simulink model "Problem_1_Part_A"  (R2018b)
settings: Solver=FixedStepAuto  StartTime=0.0  StopTime=200  FixedStep=0.01  RelTol=1e-3
InitFcn:
  | Initial_Data
StopFcn:
  | Plots_Problme_1_Part_A
values from neighbouring files (symbols this model uses):
  desired_distance = 5    [Initial_Data.m]
  K = 5    [Initial_Data.m]
  Psi0 = 0    [Initial_Data.m]
  V = 30    [Initial_Data.m]
  X0 = 500    [Initial_Data.m]
  Y0 = 0    [Initial_Data.m]
libraries: vrlib x2, simulink x1, simulink_extras x1
settings Model: Creator=User  LastModifiedBy=User

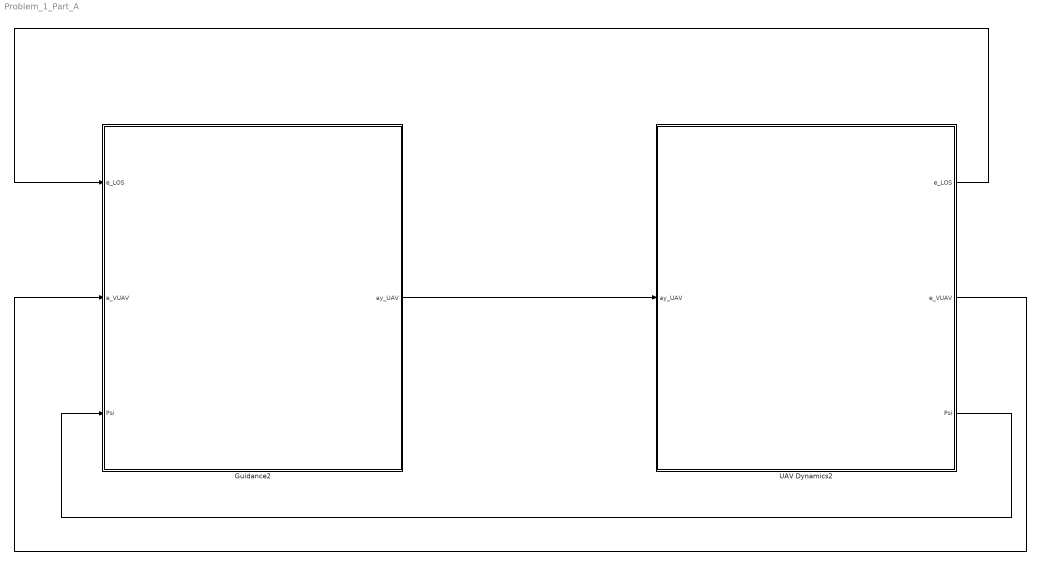
== system Problem_1_Part_A ==
  Guidance2 : Subsystem
  UAV Dynamics2 : Subsystem
  wires:
  UAV Dynamics2/2(e_VUAV) -> Guidance2/2(e_VUAV)
  UAV Dynamics2/1(e_LOS) -> Guidance2/1(e_LOS)
  UAV Dynamics2/3(Psi) -> Guidance2/3(Psi)
  Guidance2/1(ay_UAV) -> UAV Dynamics2/1(ay_UAV)

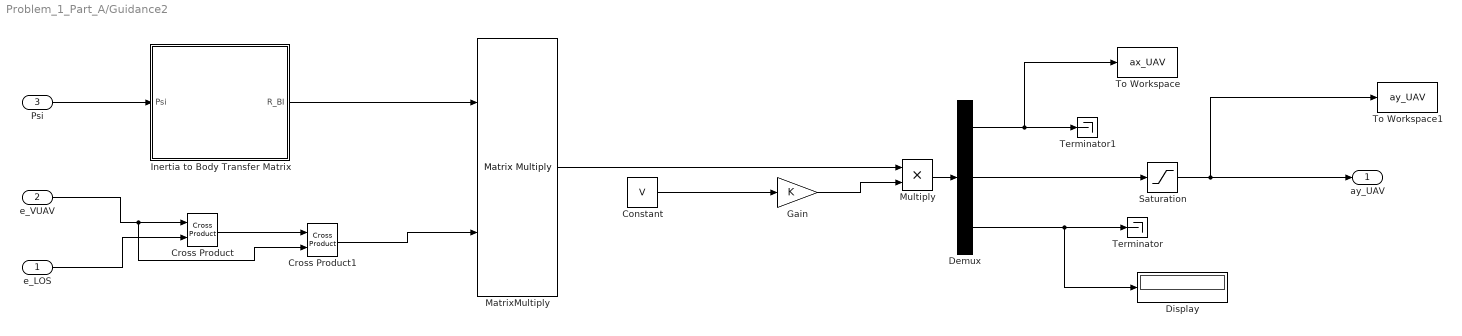
== system Problem_1_Part_A/Guidance2 ==
  e_LOS : Inport
  e_VUAV : Inport  Port=2
  Psi : Inport  Port=3
  Constant : Constant  Value=V
  Cross Product : vrlib/Utilities/Cross Product
      settings: SourceProductBaseCode=VR
  Cross Product1 : vrlib/Utilities/Cross Product
      settings: SourceProductBaseCode=VR
  Demux : Demux  Outputs=3
  Display : Display
  Gain : Gain  Gain=K
  Inertia to Body Transfer Matrix : MATLAB Function  TreatAsAtomicUnit=on
  MatrixMultiply : Product  Multiplication=Matrix(*)
  Multiply : Product
  Saturation : Saturate  UpperLimit=10  LowerLimit=-10
  Terminator : Terminator
  Terminator1 : Terminator
  To Workspace : ToWorkspace  VariableName=ax_UAV  SaveFormat=Timeseries  SampleTime=-1
  To Workspace1 : ToWorkspace  VariableName=ay_UAV  SaveFormat=Timeseries  SampleTime=-1
  ay_UAV : Outport
  wires:
  e_VUAV/1 -> Cross Product/1, Cross Product1/2
  e_LOS/1 -> Cross Product/2
  Psi/1 -> Inertia to Body Transfer Matrix/1(Psi)
  Inertia to Body Transfer Matrix/1(R_BI) -> MatrixMultiply/1
  Cross Product/1 -> Cross Product1/1
  Cross Product1/1 -> MatrixMultiply/2
  Demux/2 -> Saturation/1
  Demux/3 -> Terminator/1, Display/1
  Constant/1 -> Gain/1
  MatrixMultiply/1 -> Multiply/1
  Gain/1 -> Multiply/2
  Multiply/1 -> Demux/1
  Demux/1 -> To Workspace/1, Terminator1/1
  Saturation/1 -> To Workspace1/1, ay_UAV/1

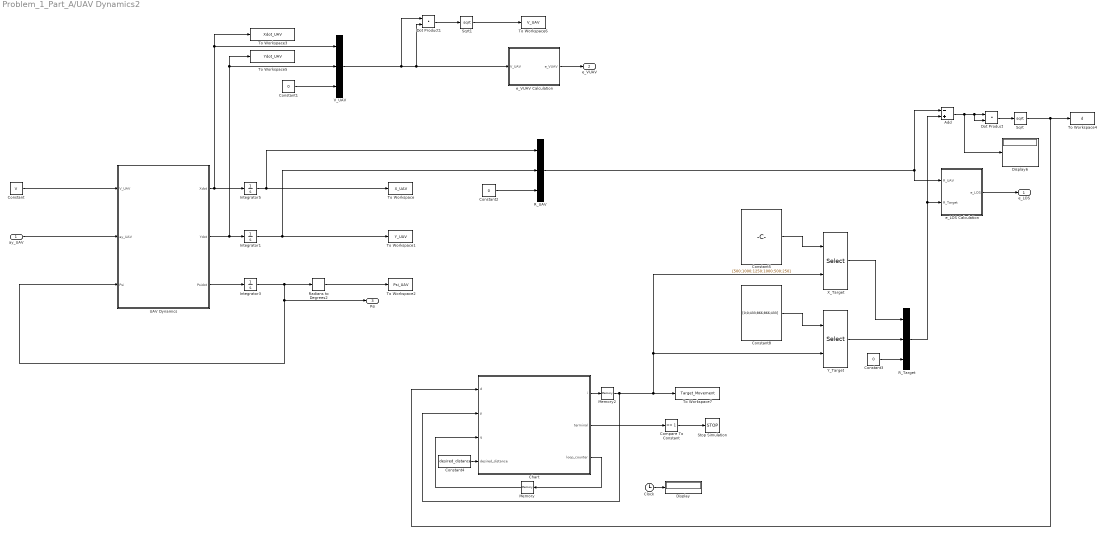
== system Problem_1_Part_A/UAV Dynamics2 ==
  ay_UAV : Inport
  Add : Sum  Inputs=-+
  Chart : Stateflow chart  TreatAsAtomicUnit=on
  Clock : Clock
  Compare To Constant : simulink/Logic and Bit Operations/Compare To Constant  relop===  const=1  OutDataTypeStr=boolean
  Constant : Constant  Value=V
  Constant1 : Constant  Value=0
  Constant2 : Constant  Value=0
  Constant3 : Constant  Value=0
  Constant4 : Constant  Value=desired_distance
  Constant5 : Constant  Value=[500;1000;1250;1000;500;250]  VectorParams1D=off
  Constant8 : Constant  Value=[0;0;433;866;866;433]  VectorParams1D=off
  Display : Display
  Display6 : Display
  Dot Product : DotProduct  InputSameDT=on  OutDataTypeStr=Inherit: Inherit via internal rule
  Dot Product1 : DotProduct  InputSameDT=on  OutDataTypeStr=Inherit: Inherit via internal rule
  Integrator1 : Integrator  InitialCondition=Y0
  Integrator3 : Integrator  InitialCondition=Psi0*pi/180
  Integrator5 : Integrator  InitialCondition=X0
  Memory : Memory  InitialCondition=1
  Memory2 : Memory  InitialCondition=2
  R_Target : Mux  Inputs=3
  R_UAV : Mux  Inputs=3
  Radians to Degrees2 : simulink_extras/Transformations/Radians to Degrees
  Sqrt : Sqrt  SaturateOnIntegerOverflow=on
  Sqrt1 : Sqrt  SaturateOnIntegerOverflow=on
  Stop Simulation : Stop
  To Workspace : ToWorkspace  VariableName=X_UAV  SaveFormat=Timeseries  SampleTime=-1
  To Workspace1 : ToWorkspace  VariableName=Y_UAV  SaveFormat=Timeseries  SampleTime=-1
  To Workspace2 : ToWorkspace  VariableName=Psi_UAV  SaveFormat=Timeseries  SampleTime=-1
  To Workspace3 : ToWorkspace  VariableName=Xdot_UAV  SaveFormat=Timeseries  SampleTime=-1
  To Workspace4 : ToWorkspace  VariableName=d  SaveFormat=Timeseries  SampleTime=-1
  To Workspace5 : ToWorkspace  VariableName=Ydot_UAV  SaveFormat=Timeseries  SampleTime=-1
  To Workspace6 : ToWorkspace  VariableName=V_UAV  SaveFormat=Timeseries  SampleTime=-1
  To Workspace7 : ToWorkspace  VariableName=Target_Movement  SaveFormat=Timeseries  SampleTime=-1
  UAV Dynamics : MATLAB Function  TreatAsAtomicUnit=on
  V_UAV : Mux  Inputs=3
  X_Target : Selector  InputPortWidth=6  IndexOptions=Index vector (port)  Indices=1  OutputSizes=2
  Y_Target : Selector  InputPortWidth=6  IndexOptions=Index vector (port)  Indices=1  OutputSizes=2
  e_LOS Calculation : MATLAB Function  TreatAsAtomicUnit=on
  e_VUAV Calculation : MATLAB Function  TreatAsAtomicUnit=on
  e_LOS : Outport
  e_VUAV : Outport  Port=2
  Psi : Outport  Port=3
  wires:
  UAV Dynamics/1(Xdot) -> Integrator5/1, To Workspace3/1, V_UAV/1
  Integrator1/1 -> To Workspace1/1, R_UAV/2
  UAV Dynamics/3(Psidot) -> Integrator3/1
  Constant2/1 -> R_UAV/3
  Constant3/1 -> R_Target/3
  R_Target/1 -> Add/2, e_LOS Calculation/2(R_Target)
  e_LOS Calculation/1(e_LOS) -> e_LOS/1
  R_UAV/1 -> e_LOS Calculation/1(R_UAV), Add/1
  e_VUAV Calculation/1(e_VUAV) -> e_VUAV/1
  Radians to Degrees2/1 -> To Workspace2/1
  Add/1 -> Display6/1, Dot Product/1, Dot Product/2
  Dot Product/1 -> Sqrt/1
  Clock/1 -> Display/1
  Memory2/1 -> Chart/2(p), Y_Target/2, X_Target/2, To Workspace7/1
  Constant8/1 -> Y_Target/1
  Y_Target/1 -> R_Target/2
  Constant5/1 -> X_Target/1
  X_Target/1 -> R_Target/1
  Chart/1(i) -> Memory2/1
  Sqrt/1 -> Chart/1(d), To Workspace4/1
  UAV Dynamics/2(Ydot) -> Integrator1/1, V_UAV/2, To Workspace5/1
  Integrator5/1 -> To Workspace/1, R_UAV/1
  ay_UAV/1 -> UAV Dynamics/2(ay_UAV)
  Constant/1 -> UAV Dynamics/1(V_UAV)
  Integrator3/1 -> Radians to Degrees2/1, UAV Dynamics/3(Psi), Psi/1
  Constant1/1 -> V_UAV/3
  V_UAV/1 -> Dot Product1/2, e_VUAV Calculation/1(V_UAV), Dot Product1/1
  Compare To Constant/1 -> Stop Simulation/1
  Chart/2(terminal) -> Compare To Constant/1
  Chart/3(loop_counter) -> Memory/1
  Memory/1 -> Chart/3(q)
  Dot Product1/1 -> Sqrt1/1
  Sqrt1/1 -> To Workspace6/1
  Constant4/1 -> Chart/4(desired_distance)

== matlab function Problem_1_Part_A/Guidance2/Inertia to Body Transfer Matrix ==
  data: R_BI output; Psi input
function R_BI = fcn(Psi)

R_Psi = [cos(Psi) sin(Psi) 0;-sin(Psi) cos(Psi) 0;0 0 1];
R_BI = R_Psi;

== stateflow chart Problem_1_Part_A/UAV Dynamics2/Chart ==
  state TargetMovement
    i = p;
    terminal = 0;
    loop_counter = q;
    if d  <  desired_distance
    i = p + 1;
    end
    if i  >  6
    i = 1;
    loop_counter = q + 1;
    end
    if i == 5 && loop_counter == 2
    terminal = 1;
    end
  (default) -> TargetMovement
  data: d input; i output; p input; terminal output; q input; loop_counter output; desired_distance input

== matlab function Problem_1_Part_A/UAV Dynamics2/UAV Dynamics ==
  data: V_UAV input; Xdot output; ay_UAV input; Ydot output; Psi input; Psidot output
function [Xdot,Ydot,Psidot]  = fcn(V_UAV,ay_UAV,Psi)

Xdot = V_UAV*cos(Psi);
Ydot = V_UAV*sin(Psi);
Psidot = ay_UAV/V_UAV;

== matlab function Problem_1_Part_A/UAV Dynamics2/e_LOS Calculation ==
  data: R_UAV input; e_LOS output; R_Target input
function e_LOS  = fcn(R_UAV,R_Target)

e_LOS = (R_Target-R_UAV)/(norm(R_Target-R_UAV));

== matlab function Problem_1_Part_A/UAV Dynamics2/e_VUAV Calculation ==
  data: V_UAV input; e_VUAV output
function e_VUAV = fcn(V_UAV)

e_VUAV = V_UAV/(norm(V_UAV));
